simulink model "operational_space_pd_w_g_comp"  (R2021b)
settings: Solver=VariableStepAuto  StartTime=0.0  StopTime=10.0  RelTol=1e-3
undefined symbols (not defined in the file): dqi, g_q, KD, KP, myRobot, qf, qi, xd
libraries: vrlib x2
settings Model: Creator=miche  LastModifiedBy=miche

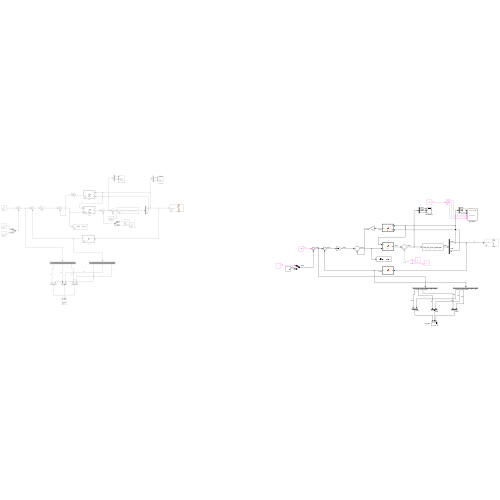
[thumbnail: Simulink's stored preview of the top-level diagram]
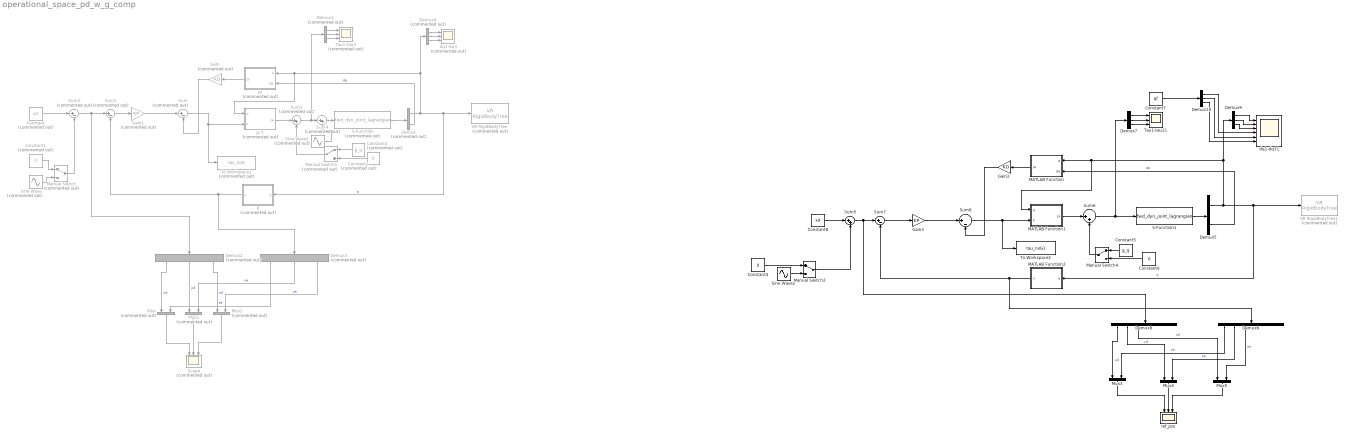
== system operational_space_pd_w_g_comp ==
  " ja T" : MATLAB Function  Commented=on  TreatAsAtomicUnit=on
  Constant : Constant  Commented=on  Value=xd
  Constant1 : Constant  Commented=on  Value=0
  Constant2 : Constant  Commented=on  Value=g_q
  Constant3 : Constant  Commented=on  Value=0
  Constant4 : Constant  Value=0
  Constant5 : Constant  Value=g_q
  Constant6 : Constant  Value=0
  Constant7 : Constant  Value=qf
  Constant8 : Constant  Value=xd
  Demux : Demux  Commented=on  Outputs=2
  Demux{1..4} (4 alike) : Demux  Commented=on  Outputs=3
  Demux10 : Demux  Outputs=3
  Demux5 : Demux  Outputs=2
  Demux6 : Demux  Outputs=6
  Demux7 : Demux  Outputs=3
  Demux8 : Demux  Outputs=6
  Demux9 : Demux  Outputs=3
  Gain : Gain  Commented=on  Gain=KD
  Gain1 : Gain  Commented=on  Gain=KP
  Gain2 : Gain  Gain=KD
  Gain3 : Gain  Gain=KP
  Ja : MATLAB Function  Commented=on  TreatAsAtomicUnit=on
  K : MATLAB Function  Commented=on  TreatAsAtomicUnit=on
  MATLAB Function : MATLAB Function  TreatAsAtomicUnit=on
  MATLAB Function1 : MATLAB Function  TreatAsAtomicUnit=on
  MATLAB Function2 : MATLAB Function  TreatAsAtomicUnit=on
  Manual Switch : ManualSwitch  Commented=on
  Manual Switch1 : ManualSwitch  Commented=on
  Manual Switch2 : ManualSwitch
  Manual Switch4 : ManualSwitch
  Mux : Mux  Commented=on  Inputs=2
  Mux1 : Mux  Commented=on  Inputs=2
  Mux2 : Mux  Commented=on  Inputs=2
  Mux3 : Mux  Inputs=2
  Mux4 : Mux  Inputs=2
  Mux5 : Mux  Inputs=2
  S-Function : S-Function  Commented=on  FunctionName=fwd_dyn_joint_lagrangian  Parameters=myRobot,qi,dqi  SFunctionDeploymentMode=off  EnableBusSupport=off
  S-Function1 : S-Function  FunctionName=fwd_dyn_joint_lagrangian  Parameters=myRobot,qi,dqi  SFunctionDeploymentMode=off  EnableBusSupport=off
  Scope : Scope  Commented=on  NumInputPorts=3
  Sine Wave : Sin  Commented=on  SampleTime=0
  Sine Wave1 : Sin  Commented=on  Amplitude=0.1  Frequency=5  SampleTime=0
  Sine Wave2 : Sin  Amplitude=0.1  SampleTime=0
  Sum : Sum  Commented=on  Inputs=|+-
  Sum1 : Sum  Commented=on  Inputs=|+-
  Sum2 : Sum  Commented=on  Inputs=|+-
  Sum3 : Sum  Commented=on  Inputs=|++
  Sum4 : Sum  Commented=on  Inputs=|++
  Sum5 : Sum  Inputs=|++
  Sum6 : Sum  Inputs=|++
  Sum7 : Sum  Inputs=|+-
  Sum8 : Sum  Inputs=|+-
  Tau1-tau3 : Scope  Commented=on  NumInputPorts=3
  Tau1-tau31 : Scope  NumInputPorts=3
  To Workspace1 : ToWorkspace  Commented=on  VariableName=tau_noG  SaveFormat=Timeseries  SampleTime=-1
  To Workspace2 : ToWorkspace  VariableName=tau_noG1  SaveFormat=Timeseries  SampleTime=-1
  VR RigidBodyTree : vrlib/VR RigidBodyTree  Commented=on  RBT=rbt  useRBT=on  Ts=-1  ForceViewerOpen=on
      settings: SourceProductBaseCode=SL
  VR RigidBodyTree1 : vrlib/VR RigidBodyTree  Commented=on  RBT=rbt  useRBT=on  Ts=-1  ForceViewerOpen=on
      settings: SourceProductBaseCode=SL
  dq1-dq3 : Scope  Commented=on  NumInputPorts=3
  dq1-dq31 : Scope  NumInputPorts=6
  ref_pos : Scope  NumInputPorts=3
  wires:
  Gain1/1 -> Sum/1
  Sum/1 -> To Workspace1/1, " ja T"/2(F)
  Gain/1 -> Sum/2
  Sum1/1 -> Gain1/1
  Constant1/1 -> Manual Switch/1
  Sine Wave/1 -> Manual Switch/2
  Constant/1 -> Sum2/1
  Manual Switch/1 -> Sum2/2
  Sum2/1 -> Demux2/1, Sum1/1
  " ja T"/1(Ja) -> Sum3/1
  Manual Switch1/1 -> Sum3/2
  Constant2/1 -> Manual Switch1/1
  Constant3/1 -> Manual Switch1/2
  S-Function/1 -> Demux/1
  Demux/1 -> K/1(q), VR RigidBodyTree/1, " ja T"/1(q), Ja/1(q), Demux4/1  "q"
  Demux/2 -> Ja/2(dq)  "dq"
  Ja/1(Ja) -> Gain/1
  K/1(x) -> Demux3/1, Sum1/2
  Demux1/1 -> Tau1-tau3/1
  Demux1/2 -> Tau1-tau3/2
  Demux1/3 -> Tau1-tau3/3
  Demux2/1 -> Mux/1  "cd"
  Demux3/1 -> Mux/2  "ze"
  Demux3/2 -> Mux1/2  "xe"
  Demux3/3 -> Mux2/2  "ye"
  Demux2/2 -> Mux1/1  "yd"
  Demux2/3 -> Mux2/1  "zd"
  Mux/1 -> Scope/1
  Mux1/1 -> Scope/2
  Mux2/1 -> Scope/3
  Demux4/2 -> dq1-dq3/2
  Demux4/3 -> dq1-dq3/3
  Demux4/1 -> dq1-dq3/1
  Sum3/1 -> Demux1/1, Sum4/1
  Sum4/1 -> S-Function/1
  Sine Wave1/1 -> Sum4/2
  MATLAB Function2/1(x) -> Demux6/1, Sum7/2
  Demux6/3 -> Mux5/2  "ze"
  Constant6/1 -> Manual Switch4/2
  Gain2/1 -> Sum8/2
  Manual Switch2/1 -> Sum5/2
  MATLAB Function/1(Ja) -> Gain2/1
  Demux6/2 -> Mux4/2  "ye"
  Sum8/1 -> MATLAB Function1/2(F), To Workspace2/1
  Constant4/1 -> Manual Switch2/1
  Demux8/2 -> Mux4/1  "yd"
  Sum7/1 -> Gain3/1
  Demux6/1 -> Mux3/2  "xe"
  S-Function1/1 -> Demux5/1
  Demux5/2 -> MATLAB Function/2(dq)  "dq"
  Demux8/3 -> Mux5/1  "zd"
  Gain3/1 -> Sum8/1
  Sine Wave2/1 -> Manual Switch2/2
  Sum5/1 -> Sum7/1, Demux8/1
  Mux4/1 -> ref_pos/2
  Constant8/1 -> Sum5/1
  Mux3/1 -> ref_pos/1
  Mux5/1 -> ref_pos/3
  Constant5/1 -> Manual Switch4/1
  Demux8/1 -> Mux3/1  "xd"
  MATLAB Function1/1(Ja) -> Sum6/1
  Sum6/1 -> Demux7/1, S-Function1/1
  Demux7/3 -> Tau1-tau31/3
  Demux7/1 -> Tau1-tau31/1
  Demux7/2 -> Tau1-tau31/2
  Demux9/1 -> dq1-dq31/1
  Demux9/2 -> dq1-dq31/2
  Demux5/1 -> MATLAB Function1/1(q), MATLAB Function/1(q), Demux9/1, VR RigidBodyTree1/1, MATLAB Function2/1(q)  "q"
  Demux9/3 -> dq1-dq31/3
  Manual Switch4/1 -> Sum6/2
  Demux10/1 -> dq1-dq31/4
  Demux10/2 -> dq1-dq31/5
  Demux10/3 -> dq1-dq31/6
  Constant7/1 -> Demux10/1

== matlab function operational_space_pd_w_g_comp/Ja ==
  data: q input; dq input; Ja output
function Ja = fcn(q, dq)
Ja = getJa(q)*dq;

== matlab function operational_space_pd_w_g_comp/ ja T ==
  data: q input; Ja output; F input
function Ja = fcn(q, F)

Ja = getJa(q)'*F;

== matlab function operational_space_pd_w_g_comp/K ==
  data: q input; x output
function x = fcn(q)
x = getK(q);

== matlab function operational_space_pd_w_g_comp/MATLAB Function ==
  data: q input size=3; Ja output; dq input
function Ja = fcn(q, dq)

Ja = getJa(q)*dq;

== matlab function operational_space_pd_w_g_comp/MATLAB Function1 ==
  data: q input size=3; Ja output size=3; F input
function Ja = fcn(q, F)

Ja = getJa(q)'*F;

== matlab function operational_space_pd_w_g_comp/MATLAB Function2 ==
  data: q input; x output
function x = fcn(q)
x = getK(q);
